simulink model "DeltaWingPlantADRC_FINAL_2018a"  (Simulink 9.1)
settings: Solver=ode45  StartTime=0.0  StopTime=100  MaxStep=0.01  RelTol=1e-3  EnableMultiTasking=on
undefined symbols (not defined in the file or in its folder): beta0, betap0, Ta, um
libraries: simulink x1
settings Model: Creator=Adam  LastModifiedBy=szymon
settings DataIOCC: LimitDataPoints=on  SignalLoggingSaveFormat=ModelDataLogs
settings OptimizationCC: InitFltsAndDblsToZero=on
settings DebuggingCC: SaveWithParameterizedLinksMsg=none  SignalResolutionControl=TryResolveAllWithWarning  SolverPrmCheckMsg=warning  MultiTaskDSMMsg=warning  MultiTaskCondExecSysMsg=none  FcnCallInpInsideContextMsg=warning
settings SFSimCC: SimUseLocalCustomCode=on
settings RTWCC: RTWUseLocalCustomCode=on
settings GRTTargetCC: TargetFcnLib=ansi_tfl_tmw.mat
settings ConfigComp: CovExternalEMLEnable=on

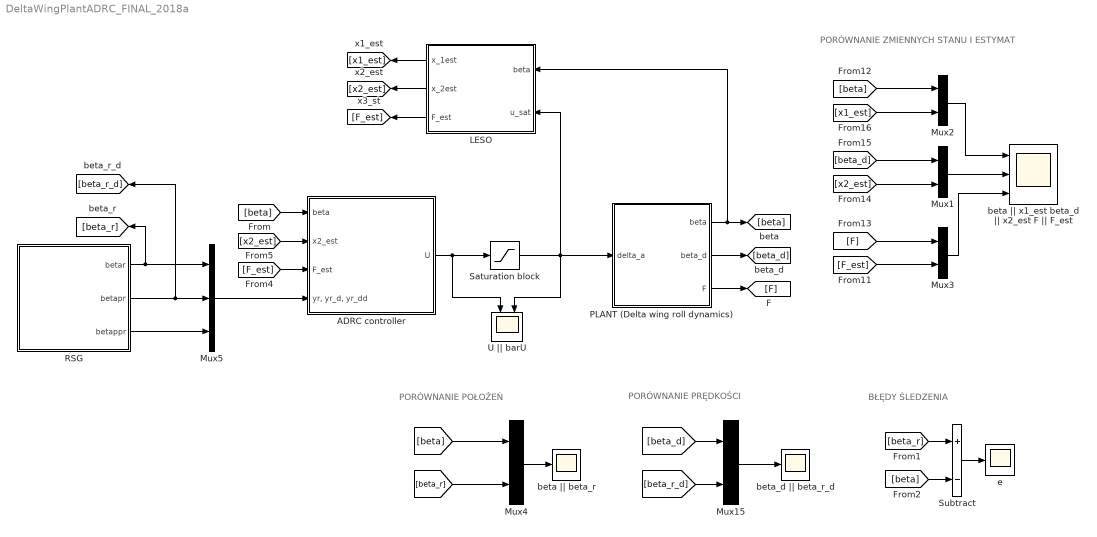
== system DeltaWingPlantADRC_FINAL_2018a ==
  note: BŁĘDY ŚLEDZENIA
  note: PORÓWNANIE ZMIENNYCH STANU I ESTYMAT
  note: PORÓWNANIE PRĘDKOŚCI
  note: PORÓWNANIE POŁOŻEŃ
  ADRC controller : Subsystem
  LESO : Subsystem
  Mux{1..4,15} (5 alike) : Mux  Inputs=2
  Mux5 : Mux  Inputs=3
  PLANT (Delta wing roll dynamics) : Subsystem
  RSG : Subsystem
  Saturation block : Saturate  UpperLimit=um  LowerLimit=-um
  Subtract : Sum  Inputs=+-
  U || barU : Scope  NumInputPorts=2
  beta || beta_r : Scope
  beta || x1_est beta_d || x2_est F || F_est : Scope  NumInputPorts=3
  beta_d || beta_r_d : Scope
  e : Scope
  wires:
  RSG/3(betappr) -> Mux5/3
  ADRC controller/1(U) -> Saturation block/1, U || barU/1
  PLANT (Delta wing roll dynamics)/1(beta) -> [beta], LESO/1(beta)
  Mux5/1 -> ADRC controller/4("yr, yr_d, yr_dd")
  Saturation block/1 -> PLANT (Delta wing roll dynamics)/1(delta_a), LESO/2(u_sat), U || barU/2
  RSG/1(betar) -> [beta_r], Mux5/1
  RSG/2(betapr) -> [beta_r_d], Mux5/2
  [beta_r] -> Subtract/1
  [beta] -> Subtract/2
  Subtract/1 -> e/1
  Mux4/1 -> beta || beta_r/1
  Mux15/1 -> beta_d || beta_r_d/1
  [beta_r_d] -> Mux15/2
  [beta_d] -> Mux15/1
  [beta_r] -> Mux4/2
  [beta] -> Mux4/1
  PLANT (Delta wing roll dynamics)/2(beta_d) -> [beta_d]
  PLANT (Delta wing roll dynamics)/3(F) -> [F]
  Mux2/1 -> beta || x1_est beta_d || x2_est F || F_est/1
  Mux1/1 -> beta || x1_est beta_d || x2_est F || F_est/2
  [beta] -> Mux2/1
  [F] -> Mux3/1
  [F_est] -> Mux3/2
  [x2_est] -> Mux1/2
  [beta_d] -> Mux1/1
  Mux3/1 -> beta || x1_est beta_d || x2_est F || F_est/3
  [x1_est] -> Mux2/2
  LESO/1(x_1est) -> [x1_est]
  LESO/2(x_2est) -> [x2_est]
  LESO/3(F_est) -> [F_est]
  [F_est] -> ADRC controller/3(F_est)
  [x2_est] -> ADRC controller/2(x2_est)
  [beta] -> ADRC controller/1(beta)

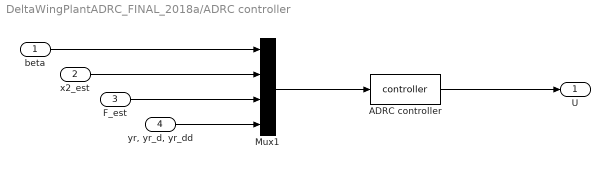
== system DeltaWingPlantADRC_FINAL_2018a/ADRC controller ==
  beta : Inport
  x2_est : Inport  Port=2
  F_est : Inport  Port=3
  "yr, yr_d, yr_dd" : Inport  Port=4
  ADRC controller : MATLABFcn  MATLABFcn=controller
  Mux1 : Mux
  U : Outport
  wires:
  Mux1/1 -> ADRC controller/1
  ADRC controller/1 -> U/1
  beta/1 -> Mux1/1
  x2_est/1 -> Mux1/2
  F_est/1 -> Mux1/3
  "yr, yr_d, yr_dd"/1 -> Mux1/4

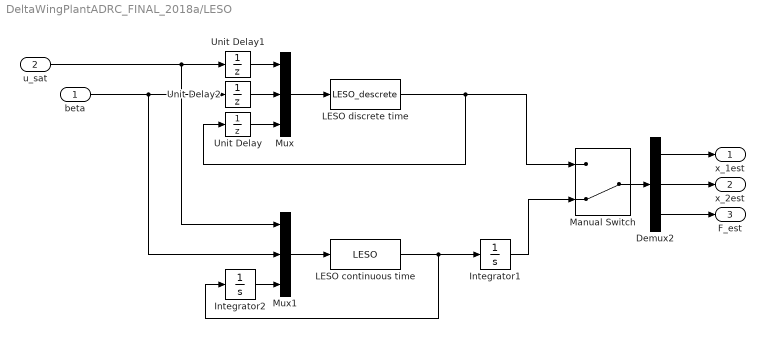
== system DeltaWingPlantADRC_FINAL_2018a/LESO ==
  beta : Inport
  u_sat : Inport  Port=2
  Demux2 : Demux  Outputs=3
  Integrator1 : Integrator  InitialCondition=[0 0 0]
  Integrator2 : Integrator  InitialCondition=[0 0 0]
  LESO continuous time : MATLABFcn  MATLABFcn=LESO  OutputDimensions=3
  LESO discrete time : MATLABFcn  MATLABFcn=LESO_descrete  OutputDimensions=3
  Manual Switch : ManualSwitch  CurrentSetting=0
  Mux : Mux  Inputs=3
  Mux1 : Mux  Inputs=3
  Unit Delay : UnitDelay  SampleTime=Ta
  Unit Delay1 : UnitDelay  SampleTime=Ta
  Unit Delay2 : UnitDelay  SampleTime=Ta
  x_1est : Outport
  x_2est : Outport  Port=2
  F_est : Outport  Port=3
  wires:
  LESO continuous time/1 -> Integrator1/1, Integrator2/1
  Mux/1 -> LESO discrete time/1
  u_sat/1 -> Mux1/1, Unit Delay1/1
  beta/1 -> Mux1/2, Unit Delay2/1
  LESO discrete time/1 -> Unit Delay/1, Manual Switch/1
  Unit Delay/1 -> Mux/3
  Mux1/1 -> LESO continuous time/1
  Integrator2/1 -> Mux1/3
  Integrator1/1 -> Manual Switch/2
  Unit Delay1/1 -> Mux/1
  Unit Delay2/1 -> Mux/2
  Demux2/3 -> F_est/1
  Demux2/1 -> x_1est/1
  Demux2/2 -> x_2est/1
  Manual Switch/1 -> Demux2/1

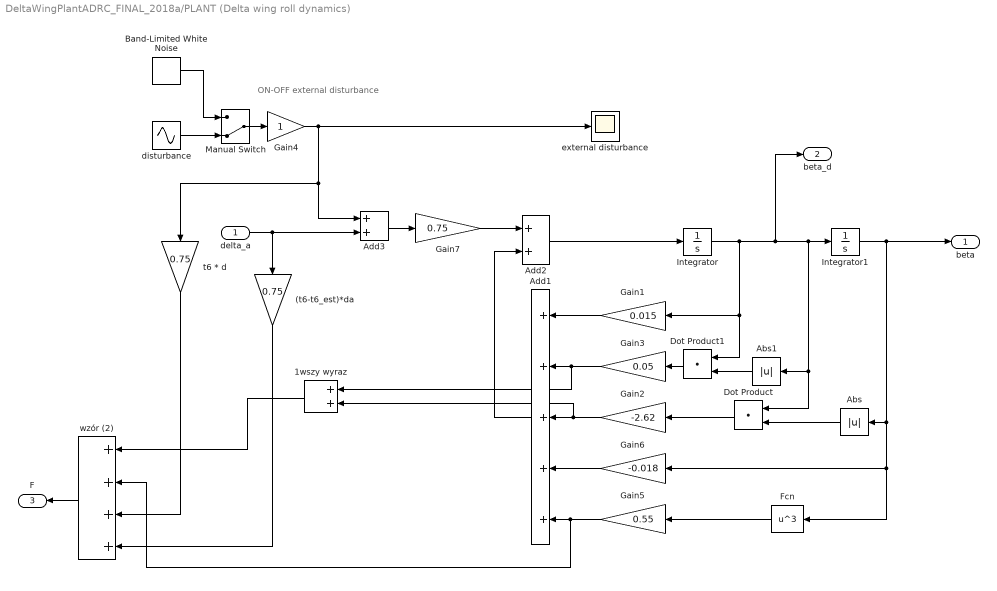
== system DeltaWingPlantADRC_FINAL_2018a/PLANT (Delta wing roll dynamics) ==
  note: ON-OFF external
      | disturbance
  delta_a : Inport
  (t6-t6_est)*da : Gain  Gain=0.75
  1wszy wyraz : Sum
  Abs : Abs
  Abs1 : Abs
  Add1 : Sum  Inputs=+++++
  Add2 : Sum
  Add3 : Sum
  Band-Limited White Noise : simulink/Sources/Band-Limited White Noise  Cov=[0.1*15]  Ts=15  seed=[23341]
  Dot Product : DotProduct  InputSameDT=on  OutDataTypeStr=Inherit: Inherit via internal rule
  Dot Product1 : DotProduct  InputSameDT=on  OutDataTypeStr=Inherit: Inherit via internal rule
  Fcn : Fcn  Expr=u^3
  Gain1 : Gain  Gain=0.015
  Gain2 : Gain  Gain=-2.62
  Gain3 : Gain  Gain=0.05
  Gain4 : Gain
  Gain5 : Gain  Gain=0.55
  Gain6 : Gain  Gain=-0.018
  Gain7 : Gain  Gain=0.75
  Integrator : Integrator  InitialCondition=betap0
  Integrator1 : Integrator  InitialCondition=beta0
  Manual Switch : ManualSwitch  CurrentSetting=0
  disturbance : Sin  Amplitude=1.5  SampleTime=0
  external disturbance : Scope
  t6 * d : Gain  Gain=0.75
  wzór (2) : Sum  Inputs=++++
  beta : Outport
  beta_d : Outport  Port=2
  F : Outport  Port=3
  wires:
  Integrator/1 -> Dot Product1/1, Gain1/1, beta_d/1, Integrator1/1, Dot Product/1, Abs1/1
  Add2/1 -> Integrator/1
  Manual Switch/1 -> Gain4/1
  Band-Limited White Noise/1 -> Manual Switch/1
  disturbance/1 -> Manual Switch/2
  Integrator1/1 -> beta/1, Gain6/1, Fcn/1, Abs/1
  Add1/1 -> Add2/2
  Fcn/1 -> Gain5/1
  Dot Product/1 -> Gain2/1
  Abs/1 -> Dot Product/2
  Abs1/1 -> Dot Product1/2
  Dot Product1/1 -> Gain3/1
  Gain1/1 -> Add1/1
  Gain3/1 -> 1wszy wyraz/1, Add1/2
  Gain2/1 -> 1wszy wyraz/2, Add1/3
  Gain6/1 -> Add1/4
  Gain5/1 -> wzór (2)/2, Add1/5
  Gain4/1 -> external disturbance/1, t6 * d/1, Add3/1
  Add3/1 -> Gain7/1
  delta_a/1 -> Add3/2, (t6-t6_est)*da/1
  Gain7/1 -> Add2/1
  1wszy wyraz/1 -> wzór (2)/1
  t6 * d/1 -> wzór (2)/3
  (t6-t6_est)*da/1 -> wzór (2)/4
  wzór (2)/1 -> F/1

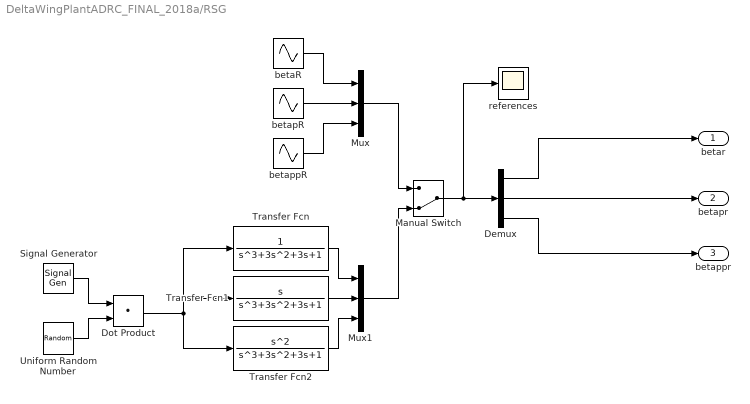
== system DeltaWingPlantADRC_FINAL_2018a/RSG ==
  Demux : Demux  Outputs=3
  Dot Product : DotProduct  InputSameDT=on  OutDataTypeStr=Inherit: Inherit via internal rule
  Manual Switch : ManualSwitch  CurrentSetting=0
  Mux : Mux  Inputs=3
  Mux1 : Mux  Inputs=3
  Signal Generator : SignalGenerator  WaveForm=square  Frequency=0.05
  Transfer Fcn : TransferFcn  Denominator=[1 3 3 1]
  Transfer Fcn1 : TransferFcn  Numerator=[1 0]  Denominator=[1 3 3 1]
  Transfer Fcn2 : TransferFcn  Numerator=[1 0 0]  Denominator=[1 3 3 1]
  Uniform Random Number : UniformRandomNumber  Minimum=-0.8*pi/2  Maximum=0.8*pi/2  SampleTime=10
  betaR : Sin  Frequency=0.5  SampleTime=0
  betapR : Sin  Amplitude=0.5  Frequency=0.5  Phase=pi/2  SampleTime=0
  betappR : Sin  Amplitude=-1*0.5*0.5  Frequency=0.5  SampleTime=0
  references : Scope
  betar : Outport
  betapr : Outport  Port=2
  betappr : Outport  Port=3
  wires:
  betaR/1 -> Mux/1
  betapR/1 -> Mux/2
  betappR/1 -> Mux/3
  Mux/1 -> Manual Switch/1
  Mux1/1 -> Manual Switch/2
  Manual Switch/1 -> Demux/1, references/1
  Demux/2 -> betapr/1
  Demux/1 -> betar/1
  Demux/3 -> betappr/1
  Transfer Fcn/1 -> Mux1/1
  Transfer Fcn1/1 -> Mux1/2
  Transfer Fcn2/1 -> Mux1/3
  Signal Generator/1 -> Dot Product/1
  Uniform Random Number/1 -> Dot Product/2
  Dot Product/1 -> Transfer Fcn1/1, Transfer Fcn/1, Transfer Fcn2/1
